simulink model "SIMULPROVA"  (R2018b)
settings: Solver=VariableStepAuto  StartTime=0.0  StopTime=10.0  RelTol=1e-3
libraries: simulink x1
settings Model: Creator=fab_d  LastModifiedBy=fab_d

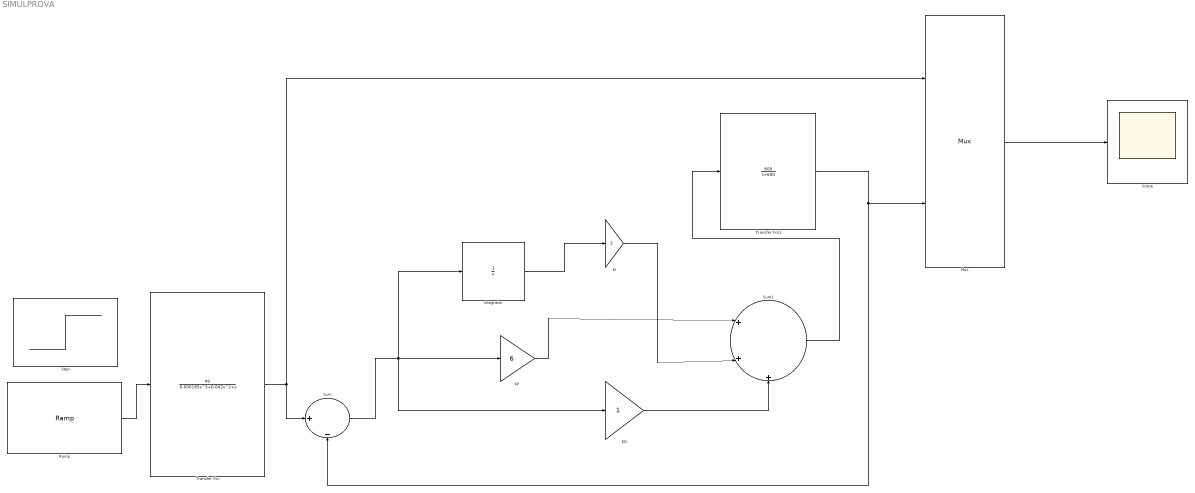
== system SIMULPROVA ==
  Integrator : Integrator
  KD : Gain
  KI : Gain  Gain=2
  KP : Gain  Gain=6
  Mux : Mux  Inputs=2
  Ramp : simulink/Sources/Ramp  slope=1  start=0  InitialOutput=0
  Scope : Scope
  Step : Step  SampleTime=0
  Sum : Sum  Inputs=|+-
  Sum1 : Sum  Inputs=|+++
  Transfer Fcn : TransferFcn  Numerator=[ 49]  Denominator="[0.000185 0.042 1 0  ]"
  Transfer Fcn1 : TransferFcn  Numerator=[ 600]  Denominator="[1 600  ]"
  wires:
  KD/1 -> Sum1/3
  KI/1 -> Sum1/2
  KP/1 -> Sum1/1
  Sum1/1 -> Transfer Fcn1/1
  Integrator/1 -> KI/1
  Transfer Fcn/1 -> Sum/1, Mux/1
  Sum/1 -> Integrator/1, KP/1, KD/1
  Ramp/1 -> Transfer Fcn/1
  Mux/1 -> Scope/1
  Transfer Fcn1/1 -> Sum/2, Mux/2
